simulink model "jellystone_v6"  (R2016b)
settings: Solver=FixedStepAuto  StartTime=0.0  StopTime=30  FixedStep=1  RelTol=1e-3
values from neighbouring files (symbols this model uses):
  acreage = 19.68    [executeModel.m]
  C0 = 2.017    [executeModel.m]    (also in project.m = 2.017+(rand-.5)*.404)
  E = x(:,1)    [executeModel.m]    (also in project.m)
  E0 = 31.217    [executeModel.m]    (also in project.m = 31.217+(rand-.5)*6.244)
  G0 = .8    (= 0.8)    [executeModel.m]    (also in project.m = .8+(rand-.5)*.16)
  graze = .492    (= 0.492)    [executeModel.m]
  W0 = .001    (= 0.001)    [executeModel.m]    (also in project.m = 0)
settings Model: Creator=thomaskennedy  LastModifiedBy=thomaskennedy
settings DebuggingCC: InitInArrayFormatMsg=none

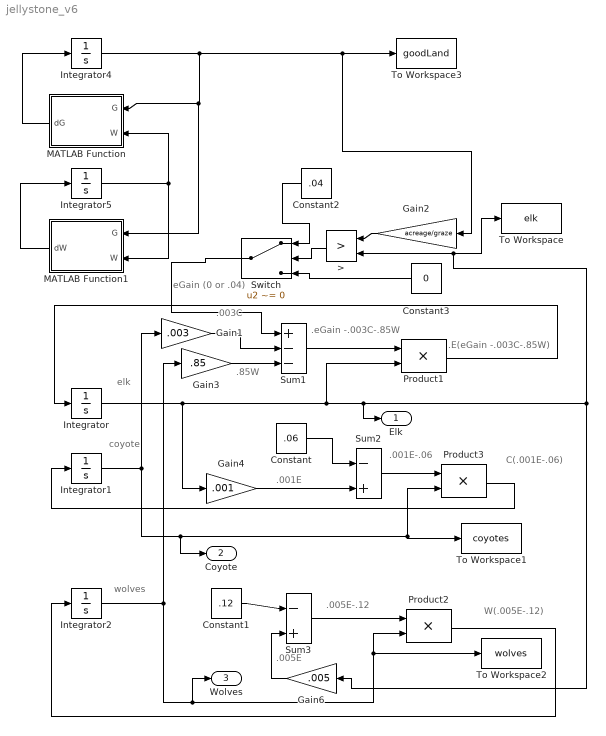
== system jellystone_v6 ==
  note: .005E
  note: elk
  note: coyote
  note: wolves
  note: .005E-.12
  note: W(.005E-.12)
  note: .001E
  note: .001E-.06
  note: C(.001E-.06)
  note: .85W
  note: .003C
  note: .eGain -.003C-.85W
  note: .E(eGain -.003C-.85W)
  note: eGain (0 or .04)
  > : RelationalOperator  Operator=>  OutDataTypeStr=boolean  RndMeth=Simplest
  Constant : Constant  Value=.06
  Constant1 : Constant  Value=.12
  Constant2 : Constant  Value=.04
  Constant3 : Constant  Value=0
  Gain1 : Gain  Gain=.003  SaturateOnIntegerOverflow=on  OutDataTypeStr=Inherit: Same as input  ParamDataTypeStr=Inherit: Same as input
  Gain2 : Gain  Gain=acreage/graze  SaturateOnIntegerOverflow=on  OutDataTypeStr=Inherit: Same as input  ParamDataTypeStr=Inherit: Same as input
  Gain3 : Gain  Gain=.85  SaturateOnIntegerOverflow=on  OutDataTypeStr=Inherit: Same as input  ParamDataTypeStr=Inherit: Same as input
  Gain4 : Gain  Gain=.001  SaturateOnIntegerOverflow=on  OutDataTypeStr=Inherit: Same as input  ParamDataTypeStr=Inherit: Same as input
  Gain6 : Gain  Gain=.005  SaturateOnIntegerOverflow=on  OutDataTypeStr=Inherit: Same as input  ParamDataTypeStr=Inherit: Same as input
  Integrator : Integrator  InitialCondition=E0
  Integrator1 : Integrator  InitialCondition=C0
  Integrator2 : Integrator  InitialCondition=W0
  Integrator4 : Integrator  InitialCondition=G0
  Integrator5 : Integrator  InitialCondition=1-G0
  MATLAB Function : MATLAB Function  TreatAsAtomicUnit=on
  MATLAB Function1 : MATLAB Function  TreatAsAtomicUnit=on
  Product1 : Product  SaturateOnIntegerOverflow=on  InputSameDT=on  OutDataTypeStr=Inherit: Same as first input
  Product2 : Product  SaturateOnIntegerOverflow=on  InputSameDT=on  OutDataTypeStr=Inherit: Same as first input
  Product3 : Product  SaturateOnIntegerOverflow=on  InputSameDT=on  OutDataTypeStr=Inherit: Same as first input
  Sum1 : Sum  Inputs=|+||-||-|  SaturateOnIntegerOverflow=on  InputSameDT=on  OutDataTypeStr=Inherit: Same as first input
  Sum2 : Sum  Inputs=|-||+|  SaturateOnIntegerOverflow=on  InputSameDT=on  OutDataTypeStr=Inherit: Same as first input
  Sum3 : Sum  Inputs=|-||+|  SaturateOnIntegerOverflow=on  InputSameDT=on  OutDataTypeStr=Inherit: Same as first input
  Switch : Switch  Criteria=u2 ~= 0  Threshold=E
  To Workspace : ToWorkspace  VariableName=elk  SampleTime=-1
  To Workspace1 : ToWorkspace  VariableName=coyotes  SampleTime=-1
  To Workspace2 : ToWorkspace  VariableName=wolves  SampleTime=-1
  To Workspace3 : ToWorkspace  VariableName=goodLand  SampleTime=-1
  Elk : Outport
  Coyote : Outport  Port=2
  Wolves : Outport  Port=3
  wires:
  Switch/1 -> Sum1/1
  Integrator1/1 -> Coyote/1, To Workspace1/1, Product3/2, Gain1/1
  Integrator/1 -> Gain4/1, Product1/2, Elk/1, >/2, To Workspace/1, Gain6/1
  Product1/1 -> Integrator/1
  Sum2/1 -> Product3/1
  Product3/1 -> Integrator1/1
  Sum1/1 -> Product1/1
  Gain1/1 -> Sum1/2
  Integrator2/1 -> Gain3/1, Wolves/1, To Workspace2/1, Product2/2
  Gain3/1 -> Sum1/3
  Constant/1 -> Sum2/1
  Gain4/1 -> Sum2/2
  Constant1/1 -> Sum3/1
  Gain6/1 -> Sum3/2
  Sum3/1 -> Product2/1
  Product2/1 -> Integrator2/1
  Integrator4/1 -> Gain2/1, To Workspace3/1, MATLAB Function1/1(G), MATLAB Function/1(G)
  Integrator5/1 -> MATLAB Function1/2(W), MATLAB Function/2(W)
  MATLAB Function1/1(dW) -> Integrator5/1
  MATLAB Function/1(dG) -> Integrator4/1
  Constant2/1 -> Switch/1
  Constant3/1 -> Switch/3
  >/1 -> Switch/2
  Gain2/1 -> >/1

== matlab function jellystone_v6/MATLAB Function1 ==
  data: G input; dW output; W input
function dW = fcn(G,W)
%Should r really be the rate of change of elk, or should it be an elk
%grazing constant?
B=0.3;
Rw=0.35;
qG=1.07;
graze=.492; %Grazing constant

dW = Rw * W * (1- W - qG*G*(1 + G/graze)/(B+G/graze));

== matlab function jellystone_v6/MATLAB Function ==
  data: G input; dG output; W input
function dG = fcn(G,W)
B=0.3;
Rg=0.27;
qW=0.6;
graze=.492; %Grazing constant
dG = Rg*G*(1-G-qW*W*(B+(G/graze))/(1+G/graze));
